simulink model "model"  (R2014a)
(part 3 of 3)

  _CN_93383685_400000_CN_149672244_400000/RConn3 -- T_149672244__Κέντρο_Υπερυψηλής_Τάσης_Τρικάλων/LConn3 -- _CN_149672244_400000_CN_85518393_400000/LConn3 -- Γραμμή_400_kV_ΚΥΤ_Αράχθου___ΚΥΤ_Τρικάλων_CN_149672244_400000_CN_140248148_400000/LConn3 -- bus123/LConn1
  _CN_93383685_400000_CN_15641949_400000/RConn1 -- G_15641949_Ατμοηλεκτρικός_Σταθμός_Αγίου_Δημητρίου/RConn1 -- _CN_55099563_400000_CN_15641949_400000/LConn1
  _CN_93383685_400000_CN_15641949_400000/RConn2 -- G_15641949_Ατμοηλεκτρικός_Σταθμός_Αγίου_Δημητρίου/RConn2 -- _CN_55099563_400000_CN_15641949_400000/LConn2
  _CN_93383685_400000_CN_15641949_400000/RConn3 -- G_15641949_Ατμοηλεκτρικός_Σταθμός_Αγίου_Δημητρίου/RConn3 -- _CN_55099563_400000_CN_15641949_400000/LConn3 -- bus124/LConn1
  _CN_93383685_400000_CN_171506480_400000/RConn1 -- T_171506480__Σταθμός_μετασχηματιστής_ρεύματος_Αμυνταίου/LConn1 -- _CN_55099563_400000_CN_171506480_400000/LConn1 -- _CN_252077527_400000_CN_171506480_400000/LConn1
  _CN_93383685_400000_CN_171506480_400000/RConn2 -- T_171506480__Σταθμός_μετασχηματιστής_ρεύματος_Αμυνταίου/LConn2 -- _CN_55099563_400000_CN_171506480_400000/LConn2 -- _CN_252077527_400000_CN_171506480_400000/LConn2
  _CN_93383685_400000_CN_171506480_400000/RConn3 -- T_171506480__Σταθμός_μετασχηματιστής_ρεύματος_Αμυνταίου/LConn3 -- _CN_55099563_400000_CN_171506480_400000/LConn3 -- bus125/LConn1 -- _CN_252077527_400000_CN_171506480_400000/LConn3
  T_249066440__/LConn1 -- _CN_93383685_400000_CN_249066440_400000/RConn1
  T_249066440__/LConn2 -- _CN_93383685_400000_CN_249066440_400000/RConn2
  _CN_93383685_400000_CN_249066440_400000/RConn3 -- T_249066440__/LConn3 -- bus126/LConn1
  Melitis___Bitola_400_kV_Line_CN_252077527_400000_CN_196633567_400000/LConn1 -- T_252077527__Κέντρο_Υπερυψηλής_Τάσης_(ΚΥΤ)_Μελίτη/LConn1 -- _CN_252077527_400000_CN_171506480_400000/RConn1
  Melitis___Bitola_400_kV_Line_CN_252077527_400000_CN_196633567_400000/LConn2 -- T_252077527__Κέντρο_Υπερυψηλής_Τάσης_(ΚΥΤ)_Μελίτη/LConn2 -- _CN_252077527_400000_CN_171506480_400000/RConn2
  Melitis___Bitola_400_kV_Line_CN_252077527_400000_CN_196633567_400000/LConn3 -- T_252077527__Κέντρο_Υπερυψηλής_Τάσης_(ΚΥΤ)_Μελίτη/LConn3 -- _CN_252077527_400000_CN_171506480_400000/RConn3 -- bus127/LConn1
  T_196633567__/LConn1 -- Melitis___Bitola_400_kV_Line_CN_252077527_400000_CN_196633567_400000/RConn1
  T_196633567__/LConn2 -- Melitis___Bitola_400_kV_Line_CN_252077527_400000_CN_196633567_400000/RConn2
  Melitis___Bitola_400_kV_Line_CN_252077527_400000_CN_196633567_400000/RConn3 -- T_196633567__/LConn3 -- bus128/LConn1
  T_140465679__Κέντρο_Υπερυψηλής_Τάσης_(ΚΥΤ)_Φιλίππων/LConn1 -- Γραμμή_400_kV_ΚΥΤ_Φιλίππων_–_ΚΥΤ_Νέας_Σάντας_CN_140465679_400000_CN_141220249_400000/LConn1
  T_140465679__Κέντρο_Υπερυψηλής_Τάσης_(ΚΥΤ)_Φιλίππων/LConn2 -- Γραμμή_400_kV_ΚΥΤ_Φιλίππων_–_ΚΥΤ_Νέας_Σάντας_CN_140465679_400000_CN_141220249_400000/LConn2
  Γραμμή_400_kV_ΚΥΤ_Φιλίππων_–_ΚΥΤ_Νέας_Σάντας_CN_140465679_400000_CN_141220249_400000/LConn3 -- T_140465679__Κέντρο_Υπερυψηλής_Τάσης_(ΚΥΤ)_Φιλίππων/LConn3 -- bus129/LConn1
  T_141220249__Κέντρο_Υπερυψηλής_Τάσης_(ΚΥΤ)_Νέας_Σάντας/LConn1 -- Γραμμή_400_kV_ΚΥΤ_Φιλίππων_–_ΚΥΤ_Νέας_Σάντας_CN_140465679_400000_CN_141220249_400000/RConn1
  T_141220249__Κέντρο_Υπερυψηλής_Τάσης_(ΚΥΤ)_Νέας_Σάντας/LConn2 -- Γραμμή_400_kV_ΚΥΤ_Φιλίππων_–_ΚΥΤ_Νέας_Σάντας_CN_140465679_400000_CN_141220249_400000/RConn2
  Γραμμή_400_kV_ΚΥΤ_Φιλίππων_–_ΚΥΤ_Νέας_Σάντας_CN_140465679_400000_CN_141220249_400000/RConn3 -- T_141220249__Κέντρο_Υπερυψηλής_Τάσης_(ΚΥΤ)_Νέας_Σάντας/LConn3 -- bus130/LConn1
  T_235044638_400000_Подстанция_Благоевград/LConn1 -- Пирин_CN_235044638_400000_CN_55099563_400000/LConn1
  T_235044638_400000_Подстанция_Благоевград/LConn2 -- Пирин_CN_235044638_400000_CN_55099563_400000/LConn2
  Пирин_CN_235044638_400000_CN_55099563_400000/LConn3 -- T_235044638_400000_Подстанция_Благоевград/LConn3 -- bus131/LConn1
  Пирин_CN_235044638_400000_CN_55099563_400000/RConn1 -- T_55099563_400000;150000_Κέντρο_Υπερυψηλής_Τάσης_Θεσσαλονίκης_(ΚΥΤ_Ωραιοκάστρου)/LConn1 -- _CN_55099563_400000_CN_15641949_400000/RConn1 -- _CN_55099563_400000_CN_171506480_400000/RConn1 -- Γραμμή_400_kV_ΚΥΤ_Θεσσαλονίκης_–_ΚΥΤ_Φιλίππων_CN_55099563_400000_CN_302950604_400000/LConn1
  Пирин_CN_235044638_400000_CN_55099563_400000/RConn2 -- T_55099563_400000;150000_Κέντρο_Υπερυψηλής_Τάσης_Θεσσαλονίκης_(ΚΥΤ_Ωραιοκάστρου)/LConn2 -- _CN_55099563_400000_CN_15641949_400000/RConn2 -- _CN_55099563_400000_CN_171506480_400000/RConn2 -- Γραμμή_400_kV_ΚΥΤ_Θεσσαλονίκης_–_ΚΥΤ_Φιλίππων_CN_55099563_400000_CN_302950604_400000/LConn2
  Пирин_CN_235044638_400000_CN_55099563_400000/RConn3 -- T_55099563_400000;150000_Κέντρο_Υπερυψηλής_Τάσης_Θεσσαλονίκης_(ΚΥΤ_Ωραιοκάστρου)/LConn3 -- _CN_55099563_400000_CN_15641949_400000/RConn3 -- _CN_55099563_400000_CN_171506480_400000/RConn3 -- bus132/LConn1 -- Γραμμή_400_kV_ΚΥΤ_Θεσσαλονίκης_–_ΚΥΤ_Φιλίππων_CN_55099563_400000_CN_302950604_400000/LConn3
  T_253903008__/LConn1 -- _CN_253903008_400000_CN_105184051_400000/LConn1
  T_253903008__/LConn2 -- _CN_253903008_400000_CN_105184051_400000/LConn2
  _CN_253903008_400000_CN_105184051_400000/LConn3 -- T_253903008__/LConn3 -- bus133/LConn1
  _CN_253903008_400000_CN_105184051_400000/RConn1 -- T_105184051_400000;150000_Κέντρο_Υπερυψηλής_Τάσης_Αχελώου/LConn1 -- Γραμμή_400_kV_ΚΥΤ_Αράχθου___ΚΥΤ_Αχελώου_CN_105184051_400000_CN_140248148_400000/LConn1
  _CN_253903008_400000_CN_105184051_400000/RConn2 -- T_105184051_400000;150000_Κέντρο_Υπερυψηλής_Τάσης_Αχελώου/LConn2 -- Γραμμή_400_kV_ΚΥΤ_Αράχθου___ΚΥΤ_Αχελώου_CN_105184051_400000_CN_140248148_400000/LConn2
  _CN_253903008_400000_CN_105184051_400000/RConn3 -- T_105184051_400000;150000_Κέντρο_Υπερυψηλής_Τάσης_Αχελώου/LConn3 -- Γραμμή_400_kV_ΚΥΤ_Αράχθου___ΚΥΤ_Αχελώου_CN_105184051_400000_CN_140248148_400000/LConn3 -- bus134/LConn1
  _CN_51408420_400000_CN_85518393_400000/LConn1 -- T_51408420__Κέντρο_Υπερυψηλής_Τάσης_Κουμουνδούρου/LConn1 -- _CN_51408420_400000_CN_85585500_400000/LConn1
  _CN_51408420_400000_CN_85518393_400000/LConn2 -- T_51408420__Κέντρο_Υπερυψηλής_Τάσης_Κουμουνδούρου/LConn2 -- _CN_51408420_400000_CN_85585500_400000/LConn2
  _CN_51408420_400000_CN_85518393_400000/LConn3 -- T_51408420__Κέντρο_Υπερυψηλής_Τάσης_Κουμουνδούρου/LConn3 -- _CN_51408420_400000_CN_85585500_400000/LConn3 -- bus135/LConn1
  _CN_51408420_400000_CN_85518393_400000/RConn1 -- T_85518393__Κέντρο_Υπερυψηλής_Τάσης_Διστόμου/LConn1 -- _CN_149672244_400000_CN_85518393_400000/RConn1 -- _CN_85526073_400000_CN_85518393_400000/LConn1
  _CN_51408420_400000_CN_85518393_400000/RConn2 -- T_85518393__Κέντρο_Υπερυψηλής_Τάσης_Διστόμου/LConn2 -- _CN_149672244_400000_CN_85518393_400000/RConn2 -- _CN_85526073_400000_CN_85518393_400000/LConn2
  _CN_51408420_400000_CN_85518393_400000/RConn3 -- T_85518393__Κέντρο_Υπερυψηλής_Τάσης_Διστόμου/LConn3 -- _CN_149672244_400000_CN_85518393_400000/RConn3 -- _CN_85526073_400000_CN_85518393_400000/LConn3 -- bus136/LConn1
  _CN_51408420_400000_CN_85585500_400000/RConn1 -- T_85585500__/LConn1 -- _CN_85526073_400000_CN_85585500_400000/LConn1
  _CN_51408420_400000_CN_85585500_400000/RConn2 -- T_85585500__/LConn2 -- _CN_85526073_400000_CN_85585500_400000/LConn2
  _CN_51408420_400000_CN_85585500_400000/RConn3 -- T_85585500__/LConn3 -- _CN_85526073_400000_CN_85585500_400000/LConn3 -- bus137/LConn1
  T_85705637_400000;150000_/LConn1 -- _CN_85705637_400000_CN_85646787_400000/LConn1
  T_85705637_400000;150000_/LConn2 -- _CN_85705637_400000_CN_85646787_400000/LConn2
  _CN_85705637_400000_CN_85646787_400000/LConn3 -- T_85705637_400000;150000_/LConn3 -- bus138/LConn1
  T_85646787__/LConn1 -- _CN_85705637_400000_CN_85646787_400000/RConn1
  T_85646787__/LConn2 -- _CN_85705637_400000_CN_85646787_400000/RConn2
  _CN_85705637_400000_CN_85646787_400000/RConn3 -- T_85646787__/LConn3 -- bus139/LConn1
  T_302950604__/LConn1 -- Γραμμή_400_kV_ΚΥΤ_Θεσσαλονίκης_–_ΚΥΤ_Φιλίππων_CN_55099563_400000_CN_302950604_400000/RConn1
  T_302950604__/LConn2 -- Γραμμή_400_kV_ΚΥΤ_Θεσσαλονίκης_–_ΚΥΤ_Φιλίππων_CN_55099563_400000_CN_302950604_400000/RConn2
  Γραμμή_400_kV_ΚΥΤ_Θεσσαλονίκης_–_ΚΥΤ_Φιλίππων_CN_55099563_400000_CN_302950604_400000/RConn3 -- T_302950604__/LConn3 -- bus140/LConn1
  Γραμμή_400_kV_ΚΥΤ_Αράχθου___ΚΥΤ_Αχελώου_CN_105184051_400000_CN_140248148_400000/RConn1 -- T_140248148__Κέντρο_Υπερυψηλής_Τάσης_Αράχθου/LConn1 -- HVDC_Italy_Greece_CN_148320055_400000_CN_140248148_400000/LConn1 -- Γραμμή_400_kV_ΚΥΤ_Αράχθου___ΚΥΤ_Τρικάλων_CN_149672244_400000_CN_140248148_400000/RConn1
  Γραμμή_400_kV_ΚΥΤ_Αράχθου___ΚΥΤ_Αχελώου_CN_105184051_400000_CN_140248148_400000/RConn2 -- T_140248148__Κέντρο_Υπερυψηλής_Τάσης_Αράχθου/LConn2 -- HVDC_Italy_Greece_CN_148320055_400000_CN_140248148_400000/LConn2 -- Γραμμή_400_kV_ΚΥΤ_Αράχθου___ΚΥΤ_Τρικάλων_CN_149672244_400000_CN_140248148_400000/RConn2
  Γραμμή_400_kV_ΚΥΤ_Αράχθου___ΚΥΤ_Αχελώου_CN_105184051_400000_CN_140248148_400000/RConn3 -- T_140248148__Κέντρο_Υπερυψηλής_Τάσης_Αράχθου/LConn3 -- HVDC_Italy_Greece_CN_148320055_400000_CN_140248148_400000/LConn3 -- bus141/LConn1 -- Γραμμή_400_kV_ΚΥΤ_Αράχθου___ΚΥΤ_Τρικάλων_CN_149672244_400000_CN_140248148_400000/RConn3
  T_148320055__/LConn1 -- HVDC_Italy_Greece_CN_148320055_400000_CN_140248148_400000/RConn1
  T_148320055__/LConn2 -- HVDC_Italy_Greece_CN_148320055_400000_CN_140248148_400000/RConn2
  HVDC_Italy_Greece_CN_148320055_400000_CN_140248148_400000/RConn3 -- T_148320055__/LConn3 -- bus142/LConn1
  _CN_85526073_400000_CN_85612093_400000/LConn1 -- T_85526073__/LConn1 -- _CN_85526073_400000_CN_86577898_400000/RConn1 -- _CN_85526073_400000_CN_85518393_400000/RConn1 -- _CN_85526073_400000_CN_85585500_400000/RConn1
  _CN_85526073_400000_CN_85612093_400000/LConn2 -- T_85526073__/LConn2 -- _CN_85526073_400000_CN_86577898_400000/RConn2 -- _CN_85526073_400000_CN_85518393_400000/RConn2 -- _CN_85526073_400000_CN_85585500_400000/RConn2
  _CN_85526073_400000_CN_85612093_400000/LConn3 -- T_85526073__/LConn3 -- _CN_85526073_400000_CN_86577898_400000/RConn3 -- _CN_85526073_400000_CN_85518393_400000/RConn3 -- _CN_85526073_400000_CN_85585500_400000/RConn3 -- bus143/LConn1
  T_85612093__/LConn1 -- _CN_85526073_400000_CN_85612093_400000/RConn1
  T_85612093__/LConn2 -- _CN_85526073_400000_CN_85612093_400000/RConn2
  _CN_85526073_400000_CN_85612093_400000/RConn3 -- T_85612093__/LConn3 -- bus144/LConn1
  T_93119207__/LConn1 -- _CN_93119207_400000_CN_86577898_400000/RConn1
  T_93119207__/LConn2 -- _CN_93119207_400000_CN_86577898_400000/RConn2
  _CN_93119207_400000_CN_86577898_400000/RConn3 -- T_93119207__/LConn3 -- bus145/LConn1
  T_134685185__/RConn1 -- L_134685185/LConn1
  T_134685185__/RConn2 -- L_134685185/LConn2
  L_134685185/LConn3 -- T_134685185__/RConn3 -- bus146/LConn1
  T_135706289__/RConn1 -- L_135706289/LConn1
  T_135706289__/RConn2 -- L_135706289/LConn2
  L_135706289/LConn3 -- T_135706289__/RConn3 -- bus147/LConn1
  T_96020492__/RConn1 -- L_96020492/LConn1
  T_96020492__/RConn2 -- L_96020492/LConn2
  L_96020492/LConn3 -- T_96020492__/RConn3 -- bus148/LConn1
  T_96314289__/RConn1 -- L_96314289/LConn1
  T_96314289__/RConn2 -- L_96314289/LConn2
  L_96314289/LConn3 -- T_96314289__/RConn3 -- bus149/LConn1
  T_140343651__/RConn1 -- L_140343651/LConn1
  T_140343651__/RConn2 -- L_140343651/LConn2
  L_140343651/LConn3 -- T_140343651__/RConn3 -- bus150/LConn1
  T_132381638__/RConn1 -- L_132381638/LConn1
  T_132381638__/RConn2 -- L_132381638/LConn2
  L_132381638/LConn3 -- T_132381638__/RConn3 -- bus151/LConn1
  T_72180968__/RConn1 -- L_72180968/LConn1
  T_72180968__/RConn2 -- L_72180968/LConn2
  L_72180968/LConn3 -- T_72180968__/RConn3 -- bus152/LConn1
  T_92611161__/RConn1 -- L_92611161/LConn1
  T_92611161__/RConn2 -- L_92611161/LConn2
  L_92611161/LConn3 -- T_92611161__/RConn3 -- bus153/LConn1
  T_92611154__/RConn1 -- L_92611154/LConn1
  T_92611154__/RConn2 -- L_92611154/LConn2
  L_92611154/LConn3 -- T_92611154__/RConn3 -- bus154/LConn1
  T_249407518__/RConn1 -- L_249407518/LConn1
  T_249407518__/RConn2 -- L_249407518/LConn2
  L_249407518/LConn3 -- T_249407518__/RConn3 -- bus155/LConn1
  T_196753738__/RConn1 -- L_196753738/LConn1
  T_196753738__/RConn2 -- L_196753738/LConn2
  L_196753738/LConn3 -- T_196753738__/RConn3 -- bus156/LConn1
  T_249407519__/RConn1 -- L_249407519/LConn1
  T_249407519__/RConn2 -- L_249407519/LConn2
  L_249407519/LConn3 -- T_249407519__/RConn3 -- bus157/LConn1
  T_249407528__/RConn1 -- L_249407528/LConn1
  T_249407528__/RConn2 -- L_249407528/LConn2
  L_249407528/LConn3 -- T_249407528__/RConn3 -- bus158/LConn1
  T_95989793__/RConn1 -- L_95989793/LConn1
  T_95989793__/RConn2 -- L_95989793/LConn2
  L_95989793/LConn3 -- T_95989793__/RConn3 -- bus159/LConn1
  T_92352843__/RConn1 -- L_92352843/LConn1
  T_92352843__/RConn2 -- L_92352843/LConn2
  L_92352843/LConn3 -- T_92352843__/RConn3 -- bus160/LConn1
  T_134935126__/RConn1 -- L_134935126/LConn1
  T_134935126__/RConn2 -- L_134935126/LConn2
  L_134935126/LConn3 -- T_134935126__/RConn3 -- bus161/LConn1
  T_93645374__/RConn1 -- L_93645374/LConn1
  T_93645374__/RConn2 -- L_93645374/LConn2
  L_93645374/LConn3 -- T_93645374__/RConn3 -- bus162/LConn1
  T_93702884__/RConn1 -- L_93702884/LConn1
  T_93702884__/RConn2 -- L_93702884/LConn2
  L_93702884/LConn3 -- T_93702884__/RConn3 -- bus163/LConn1
  T_134819995__/RConn1 -- L_134819995/LConn1
  T_134819995__/RConn2 -- L_134819995/LConn2
  L_134819995/LConn3 -- T_134819995__/RConn3 -- bus164/LConn1
  T_142656551__/RConn1 -- L_142656551/LConn1
  T_142656551__/RConn2 -- L_142656551/LConn2
  L_142656551/LConn3 -- T_142656551__/RConn3 -- bus165/LConn1
  T_140637735__/RConn1 -- L_140637735/LConn1
  T_140637735__/RConn2 -- L_140637735/LConn2
  L_140637735/LConn3 -- T_140637735__/RConn3 -- bus166/LConn1
  T_140724364__/RConn1 -- L_140724364/LConn1
  T_140724364__/RConn2 -- L_140724364/LConn2
  L_140724364/LConn3 -- T_140724364__/RConn3 -- bus167/LConn1
  T_140890157__/RConn1 -- L_140890157/LConn1
  T_140890157__/RConn2 -- L_140890157/LConn2
  L_140890157/LConn3 -- T_140890157__/RConn3 -- bus168/LConn1
  T_135463990__/RConn1 -- L_135463990/LConn1
  T_135463990__/RConn2 -- L_135463990/LConn2
  L_135463990/LConn3 -- T_135463990__/RConn3 -- bus169/LConn1
  T_93061390__/RConn1 -- L_93061390/LConn1
  T_93061390__/RConn2 -- L_93061390/LConn2
  L_93061390/LConn3 -- T_93061390__/RConn3 -- bus170/LConn1
  T_135177715__ΥΠΟΣΤΑΘΜΟΣ__Δ_Ε_Η_/RConn1 -- L_135177715/LConn1
  T_135177715__ΥΠΟΣΤΑΘΜΟΣ__Δ_Ε_Η_/RConn2 -- L_135177715/LConn2
  L_135177715/LConn3 -- T_135177715__ΥΠΟΣΤΑΘΜΟΣ__Δ_Ε_Η_/RConn3 -- bus171/LConn1
  T_128088635__/RConn1 -- L_128088635/LConn1
  T_128088635__/RConn2 -- L_128088635/LConn2
  L_128088635/LConn3 -- T_128088635__/RConn3 -- bus172/LConn1
  T_93073613__/RConn1 -- L_93073613/LConn1
  T_93073613__/RConn2 -- L_93073613/LConn2
  L_93073613/LConn3 -- T_93073613__/RConn3 -- bus173/LConn1
  T_136549173__/RConn1 -- L_136549173/LConn1
  T_136549173__/RConn2 -- L_136549173/LConn2
  L_136549173/LConn3 -- T_136549173__/RConn3 -- bus174/LConn1
  T_248889404__/RConn1 -- L_248889404/LConn1
  T_248889404__/RConn2 -- L_248889404/LConn2
  L_248889404/LConn3 -- T_248889404__/RConn3 -- bus175/LConn1
  T_136549175__/RConn1 -- L_136549175/LConn1
  T_136549175__/RConn2 -- L_136549175/LConn2
  L_136549175/LConn3 -- T_136549175__/RConn3 -- bus176/LConn1
  T_136543640__/RConn1 -- L_136543640/LConn1
  T_136543640__/RConn2 -- L_136543640/LConn2
  L_136543640/LConn3 -- T_136543640__/RConn3 -- bus177/LConn1
  T_134630651__/RConn1 -- L_134630651/LConn1
  T_134630651__/RConn2 -- L_134630651/LConn2
  L_134630651/LConn3 -- T_134630651__/RConn3 -- bus178/LConn1
  T_93583004__/RConn1 -- L_93583004/LConn1
  T_93583004__/RConn2 -- L_93583004/LConn2
  L_93583004/LConn3 -- T_93583004__/RConn3 -- bus179/LConn1
  T_86466243__Υ_Σ_Ανατολής/RConn1 -- L_86466243/LConn1
  T_86466243__Υ_Σ_Ανατολής/RConn2 -- L_86466243/LConn2
  L_86466243/LConn3 -- T_86466243__Υ_Σ_Ανατολής/RConn3 -- bus180/LConn1
  T_143622720__/RConn1 -- L_143622720/LConn1
  T_143622720__/RConn2 -- L_143622720/LConn2
  L_143622720/LConn3 -- T_143622720__/RConn3 -- bus181/LConn1
  T_120740424__/RConn1 -- L_120740424/LConn1
  T_120740424__/RConn2 -- L_120740424/LConn2
  L_120740424/LConn3 -- T_120740424__/RConn3 -- bus182/LConn1
  T_128799211__/RConn1 -- L_128799211/LConn1
  T_128799211__/RConn2 -- L_128799211/LConn2
  L_128799211/LConn3 -- T_128799211__/RConn3 -- bus183/LConn1
  T_141764450__/RConn1 -- L_141764450/LConn1
  T_141764450__/RConn2 -- L_141764450/LConn2
  L_141764450/LConn3 -- T_141764450__/RConn3 -- bus184/LConn1
  T_92611147__/RConn1 -- L_92611147/LConn1
  T_92611147__/RConn2 -- L_92611147/LConn2
  L_92611147/LConn3 -- T_92611147__/RConn3 -- bus185/LConn1
  T_249414224__/RConn1 -- L_249414224/LConn1
  T_249414224__/RConn2 -- L_249414224/LConn2
  L_249414224/LConn3 -- T_249414224__/RConn3 -- bus186/LConn1
  T_120913153__/RConn1 -- L_120913153/LConn1
  T_120913153__/RConn2 -- L_120913153/LConn2
  L_120913153/LConn3 -- T_120913153__/RConn3 -- bus187/LConn1
  T_142066771__/RConn1 -- L_142066771/LConn1
  T_142066771__/RConn2 -- L_142066771/LConn2
  L_142066771/LConn3 -- T_142066771__/RConn3 -- bus188/LConn1
  T_142066784__/RConn1 -- L_142066784/LConn1
  T_142066784__/RConn2 -- L_142066784/LConn2
  L_142066784/LConn3 -- T_142066784__/RConn3 -- bus189/LConn1
  T_178234508__/RConn1 -- L_178234508/LConn1
  T_178234508__/RConn2 -- L_178234508/LConn2
  L_178234508/LConn3 -- T_178234508__/RConn3 -- bus190/LConn1
  T_143520210__/RConn1 -- L_143520210/LConn1
  T_143520210__/RConn2 -- L_143520210/LConn2
  L_143520210/LConn3 -- T_143520210__/RConn3 -- bus191/LConn1
  T_93085785__/RConn1 -- L_93085785/LConn1
  T_93085785__/RConn2 -- L_93085785/LConn2
  L_93085785/LConn3 -- T_93085785__/RConn3 -- bus192/LConn1
  T_93085804__/RConn1 -- L_93085804/LConn1
  T_93085804__/RConn2 -- L_93085804/LConn2
  L_93085804/LConn3 -- T_93085804__/RConn3 -- bus193/LConn1
  T_279628389__/RConn1 -- L_279628389/LConn1
  T_279628389__/RConn2 -- L_279628389/LConn2
  L_279628389/LConn3 -- T_279628389__/RConn3 -- bus194/LConn1
  T_148899598__/RConn1 -- L_148899598/LConn1
  T_148899598__/RConn2 -- L_148899598/LConn2
  L_148899598/LConn3 -- T_148899598__/RConn3 -- bus195/LConn1
  T_149026603__/RConn1 -- L_149026603/LConn1
  T_149026603__/RConn2 -- L_149026603/LConn2
  L_149026603/LConn3 -- T_149026603__/RConn3 -- bus196/LConn1
  T_141514344__/RConn1 -- L_141514344/LConn1
  T_141514344__/RConn2 -- L_141514344/LConn2
  L_141514344/LConn3 -- T_141514344__/RConn3 -- bus197/LConn1
  T_148881241__/RConn1 -- L_148881241/LConn1
  T_148881241__/RConn2 -- L_148881241/LConn2
  L_148881241/LConn3 -- T_148881241__/RConn3 -- bus198/LConn1
  T_129452806__/RConn1 -- L_129452806/LConn1
  T_129452806__/RConn2 -- L_129452806/LConn2
  L_129452806/LConn3 -- T_129452806__/RConn3 -- bus199/LConn1
  T_252802673__/RConn1 -- L_252802673/LConn1
  T_252802673__/RConn2 -- L_252802673/LConn2
  L_252802673/LConn3 -- T_252802673__/RConn3 -- bus200/LConn1
  T_142180032__/RConn1 -- L_142180032/LConn1
  T_142180032__/RConn2 -- L_142180032/LConn2
  L_142180032/LConn3 -- T_142180032__/RConn3 -- bus201/LConn1
  T_142174863__/RConn1 -- L_142174863/LConn1
  T_142174863__/RConn2 -- L_142174863/LConn2
  L_142174863/LConn3 -- T_142174863__/RConn3 -- bus202/LConn1
  T_128870336__/RConn1 -- L_128870336/LConn1
  T_128870336__/RConn2 -- L_128870336/LConn2
  L_128870336/LConn3 -- T_128870336__/RConn3 -- bus203/LConn1
  T_148320053__/RConn1 -- L_148320053/LConn1
  T_148320053__/RConn2 -- L_148320053/LConn2
  L_148320053/LConn3 -- T_148320053__/RConn3 -- bus204/LConn1
  T_141685890__/RConn1 -- L_141685890/LConn1
  T_141685890__/RConn2 -- L_141685890/LConn2
  L_141685890/LConn3 -- T_141685890__/RConn3 -- bus205/LConn1
  T_93885376__/RConn1 -- L_93885376/LConn1
  T_93885376__/RConn2 -- L_93885376/LConn2
  L_93885376/LConn3 -- T_93885376__/RConn3 -- bus206/LConn1
  T_141685891__/RConn1 -- L_141685891/LConn1
  T_141685891__/RConn2 -- L_141685891/LConn2
  L_141685891/LConn3 -- T_141685891__/RConn3 -- bus207/LConn1
  T_141113249__/RConn1 -- L_141113249/LConn1
  T_141113249__/RConn2 -- L_141113249/LConn2
  L_141113249/LConn3 -- T_141113249__/RConn3 -- bus208/LConn1
  T_141533837__/RConn1 -- L_141533837/LConn1
  T_141533837__/RConn2 -- L_141533837/LConn2
  L_141533837/LConn3 -- T_141533837__/RConn3 -- bus209/LConn1
  T_141533838__/RConn1 -- L_141533838/LConn1
  T_141533838__/RConn2 -- L_141533838/LConn2
  L_141533838/LConn3 -- T_141533838__/RConn3 -- bus210/LConn1
  T_253912195__/RConn1 -- L_253912195/LConn1
  T_253912195__/RConn2 -- L_253912195/LConn2
  L_253912195/LConn3 -- T_253912195__/RConn3 -- bus211/LConn1
  T_149468818__/RConn1 -- L_149468818/LConn1
  T_149468818__/RConn2 -- L_149468818/LConn2
  L_149468818/LConn3 -- T_149468818__/RConn3 -- bus212/LConn1
  T_149481032__/RConn1 -- L_149481032/LConn1
  T_149481032__/RConn2 -- L_149481032/LConn2
  L_149481032/LConn3 -- T_149481032__/RConn3 -- bus213/LConn1
  T_254347424__/RConn1 -- L_254347424/LConn1
  T_254347424__/RConn2 -- L_254347424/LConn2
  L_254347424/LConn3 -- T_254347424__/RConn3 -- bus214/LConn1
  T_136370140__/RConn1 -- L_136370140/LConn1
  T_136370140__/RConn2 -- L_136370140/LConn2
  L_136370140/LConn3 -- T_136370140__/RConn3 -- bus215/LConn1
  T_159413454__/RConn1 -- L_159413454/LConn1
  T_159413454__/RConn2 -- L_159413454/LConn2
  L_159413454/LConn3 -- T_159413454__/RConn3 -- bus216/LConn1
  T_92508649__/RConn1 -- L_92508649/LConn1
  T_92508649__/RConn2 -- L_92508649/LConn2
  L_92508649/LConn3 -- T_92508649__/RConn3 -- bus217/LConn1
  T_92508651__Υποσταθμός_Δόξας/RConn1 -- L_92508651/LConn1
  T_92508651__Υποσταθμός_Δόξας/RConn2 -- L_92508651/LConn2
  L_92508651/LConn3 -- T_92508651__Υποσταθμός_Δόξας/RConn3 -- bus218/LConn1
  T_141029834__/RConn1 -- L_141029834/LConn1
  T_141029834__/RConn2 -- L_141029834/LConn2
  L_141029834/LConn3 -- T_141029834__/RConn3 -- bus219/LConn1
  T_249407521__Υδροηλεκτρικό_Εργοστάσιο_Λάδωνα/RConn1 -- L_249407521/LConn1
  T_249407521__Υδροηλεκτρικό_Εργοστάσιο_Λάδωνα/RConn2 -- L_249407521/LConn2
  L_249407521/LConn3 -- T_249407521__Υδροηλεκτρικό_Εργοστάσιο_Λάδωνα/RConn3 -- bus220/LConn1
  T_159413450__/RConn1 -- L_159413450/LConn1
  T_159413450__/RConn2 -- L_159413450/LConn2
  L_159413450/LConn3 -- T_159413450__/RConn3 -- bus221/LConn1
  T_159413451__/RConn1 -- L_159413451/LConn1
  T_159413451__/RConn2 -- L_159413451/LConn2
  L_159413451/LConn3 -- T_159413451__/RConn3 -- bus222/LConn1
  T_254057189__/RConn1 -- L_254057189/LConn1
  T_254057189__/RConn2 -- L_254057189/LConn2
  L_254057189/LConn3 -- T_254057189__/RConn3 -- bus223/LConn1
  T_135266022__/RConn1 -- L_135266022/LConn1
  T_135266022__/RConn2 -- L_135266022/LConn2
  L_135266022/LConn3 -- T_135266022__/RConn3 -- bus224/LConn1
  T_96040682__/RConn1 -- L_96040682/LConn1
  T_96040682__/RConn2 -- L_96040682/LConn2
  L_96040682/LConn3 -- T_96040682__/RConn3 -- bus225/LConn1
  T_129452812__/RConn1 -- L_129452812/LConn1
  T_129452812__/RConn2 -- L_129452812/LConn2
  L_129452812/LConn3 -- T_129452812__/RConn3 -- bus226/LConn1
  T_136450393__/RConn1 -- L_136450393/LConn1
  T_136450393__/RConn2 -- L_136450393/LConn2
  L_136450393/LConn3 -- T_136450393__/RConn3 -- bus227/LConn1
  T_249108719__/RConn1 -- L_249108719/LConn1
  T_249108719__/RConn2 -- L_249108719/LConn2
  L_249108719/LConn3 -- T_249108719__/RConn3 -- bus228/LConn1
  T_96040696__/RConn1 -- L_96040696/LConn1
  T_96040696__/RConn2 -- L_96040696/LConn2
  L_96040696/LConn3 -- T_96040696__/RConn3 -- bus229/LConn1
  T_96314286__/RConn1 -- L_96314286/LConn1
  T_96314286__/RConn2 -- L_96314286/LConn2
  L_96314286/LConn3 -- T_96314286__/RConn3 -- bus230/LConn1
  T_96314284__/RConn1 -- L_96314284/LConn1
  T_96314284__/RConn2 -- L_96314284/LConn2
  L_96314284/LConn3 -- T_96314284__/RConn3 -- bus231/LConn1
  T_149922042__/RConn1 -- L_149922042/LConn1
  T_149922042__/RConn2 -- L_149922042/LConn2
  L_149922042/LConn3 -- T_149922042__/RConn3 -- bus232/LConn1
  T_149922043__/RConn1 -- L_149922043/LConn1
  T_149922043__/RConn2 -- L_149922043/LConn2
  L_149922043/LConn3 -- T_149922043__/RConn3 -- bus233/LConn1
  T_148899588__/RConn1 -- L_148899588/LConn1
  T_148899588__/RConn2 -- L_148899588/LConn2
  L_148899588/LConn3 -- T_148899588__/RConn3 -- bus234/LConn1
  T_149069221__/RConn1 -- L_149069221/LConn1
  T_149069221__/RConn2 -- L_149069221/LConn2
  L_149069221/LConn3 -- T_149069221__/RConn3 -- bus235/LConn1
  T_93173562__/RConn1 -- L_93173562/LConn1
  T_93173562__/RConn2 -- L_93173562/LConn2
  L_93173562/LConn3 -- T_93173562__/RConn3 -- bus236/LConn1
  T_129452815__/RConn1 -- L_129452815/LConn1
  T_129452815__/RConn2 -- L_129452815/LConn2
  L_129452815/LConn3 -- T_129452815__/RConn3 -- bus237/LConn1
  T_148899591__/RConn1 -- L_148899591/LConn1
  T_148899591__/RConn2 -- L_148899591/LConn2
  L_148899591/LConn3 -- T_148899591__/RConn3 -- bus238/LConn1
  T_93061385__/RConn1 -- L_93061385/LConn1
  T_93061385__/RConn2 -- L_93061385/LConn2
  L_93061385/LConn3 -- T_93061385__/RConn3 -- bus239/LConn1
  T_115027244__/RConn1 -- L_115027244/LConn1
  T_115027244__/RConn2 -- L_115027244/LConn2
  L_115027244/LConn3 -- T_115027244__/RConn3 -- bus240/LConn1
  T_149026599__Σταθμός_Ηλεκτρικού_Ρεύματος_του_Άγρα/RConn1 -- L_149026599/LConn1
  T_149026599__Σταθμός_Ηλεκτρικού_Ρεύματος_του_Άγρα/RConn2 -- L_149026599/LConn2
  L_149026599/LConn3 -- T_149026599__Σταθμός_Ηλεκτρικού_Ρεύματος_του_Άγρα/RConn3 -- bus241/LConn1
  T_93368205__/RConn1 -- L_93368205/LConn1
  T_93368205__/RConn2 -- L_93368205/LConn2
  L_93368205/LConn3 -- T_93368205__/RConn3 -- bus242/LConn1
  T_149672242__/RConn1 -- L_149672242/LConn1
  T_149672242__/RConn2 -- L_149672242/LConn2
  L_149672242/LConn3 -- T_149672242__/RConn3 -- bus243/LConn1
  T_136549181__/RConn1 -- L_136549181/LConn1
  T_136549181__/RConn2 -- L_136549181/LConn2
  L_136549181/LConn3 -- T_136549181__/RConn3 -- bus244/LConn1
  T_96759614__/RConn1 -- L_96759614/LConn1
  T_96759614__/RConn2 -- L_96759614/LConn2
  L_96759614/LConn3 -- T_96759614__/RConn3 -- bus245/LConn1
  T_93906290__/RConn1 -- L_93906290/LConn1
  T_93906290__/RConn2 -- L_93906290/LConn2
  L_93906290/LConn3 -- T_93906290__/RConn3 -- bus246/LConn1
  T_93906327__/RConn1 -- L_93906327/LConn1
  T_93906327__/RConn2 -- L_93906327/LConn2
  L_93906327/LConn3 -- T_93906327__/RConn3 -- bus247/LConn1
  T_136369149__/RConn1 -- L_136369149/LConn1
  T_136369149__/RConn2 -- L_136369149/LConn2
  L_136369149/LConn3 -- T_136369149__/RConn3 -- bus248/LConn1
  T_219975140__/RConn1 -- L_219975140/LConn1
  T_219975140__/RConn2 -- L_219975140/LConn2
  L_219975140/LConn3 -- T_219975140__/RConn3 -- bus249/LConn1
  T_249066440__/RConn1 -- L_249066440/LConn1
  T_249066440__/RConn2 -- L_249066440/LConn2
  L_249066440/LConn3 -- T_249066440__/RConn3 -- bus250/LConn1
  T_252077527__Κέντρο_Υπερυψηλής_Τάσης_(ΚΥΤ)_Μελίτη/RConn1 -- L_252077527/LConn1
  T_252077527__Κέντρο_Υπερυψηλής_Τάσης_(ΚΥΤ)_Μελίτη/RConn2 -- L_252077527/LConn2
  L_252077527/LConn3 -- T_252077527__Κέντρο_Υπερυψηλής_Τάσης_(ΚΥΤ)_Μελίτη/RConn3 -- bus251/LConn1
  T_196633567__/RConn1 -- L_196633567/LConn1
  T_196633567__/RConn2 -- L_196633567/LConn2
  L_196633567/LConn3 -- T_196633567__/RConn3 -- bus252/LConn1
  T_141220249__Κέντρο_Υπερυψηλής_Τάσης_(ΚΥΤ)_Νέας_Σάντας/RConn1 -- L_141220249/LConn1
  T_141220249__Κέντρο_Υπερυψηλής_Τάσης_(ΚΥΤ)_Νέας_Σάντας/RConn2 -- L_141220249/LConn2
  L_141220249/LConn3 -- T_141220249__Κέντρο_Υπερυψηλής_Τάσης_(ΚΥΤ)_Νέας_Σάντας/RConn3 -- bus253/LConn1
  T_235044638_400000_Подстанция_Благоевград/RConn1 -- L_235044638/LConn1
  T_235044638_400000_Подстанция_Благоевград/RConn2 -- L_235044638/LConn2
  L_235044638/LConn3 -- T_235044638_400000_Подстанция_Благоевград/RConn3 -- bus254/LConn1
  T_253903008__/RConn1 -- L_253903008/LConn1
  T_253903008__/RConn2 -- L_253903008/LConn2
  L_253903008/LConn3 -- T_253903008__/RConn3 -- bus255/LConn1
  T_85585500__/RConn1 -- L_85585500/LConn1
  T_85585500__/RConn2 -- L_85585500/LConn2
  L_85585500/LConn3 -- T_85585500__/RConn3 -- bus256/LConn1
  T_85705637_400000;150000_/RConn1 -- L_85705637/LConn1
  T_85705637_400000;150000_/RConn2 -- L_85705637/LConn2
  L_85705637/LConn3 -- T_85705637_400000;150000_/RConn3 -- bus257/LConn1
  T_302950604__/RConn1 -- L_302950604/LConn1
  T_302950604__/RConn2 -- L_302950604/LConn2
  L_302950604/LConn3 -- T_302950604__/RConn3 -- bus258/LConn1
  T_148320055__/RConn1 -- L_148320055/LConn1
  T_148320055__/RConn2 -- L_148320055/LConn2
  L_148320055/LConn3 -- T_148320055__/RConn3 -- bus259/LConn1
  T_93119207__/RConn1 -- L_93119207/LConn1
  T_93119207__/RConn2 -- L_93119207/LConn2
  L_93119207/LConn3 -- T_93119207__/RConn3 -- bus260/LConn1
